simulink subsystem "Day2_Scenario_1"  (R2024a)
settings: Solver=VariableStepAuto  StartTime=0.0  StopTime=10.0  RelTol=1e-3
libraries: CarMaker4SL x2
settings Model: Creator=junhyung.cha  LastModifiedBy=User

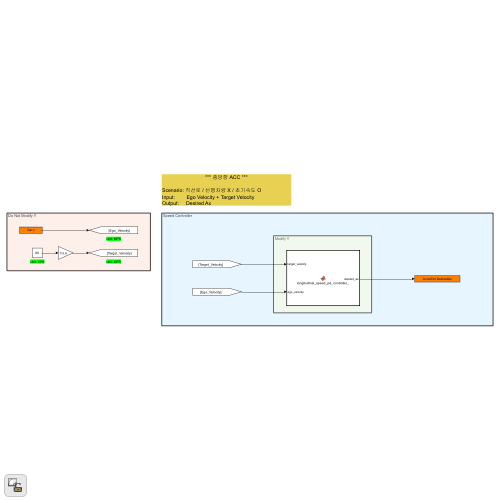
[thumbnail: Simulink's stored preview of the top-level diagram]
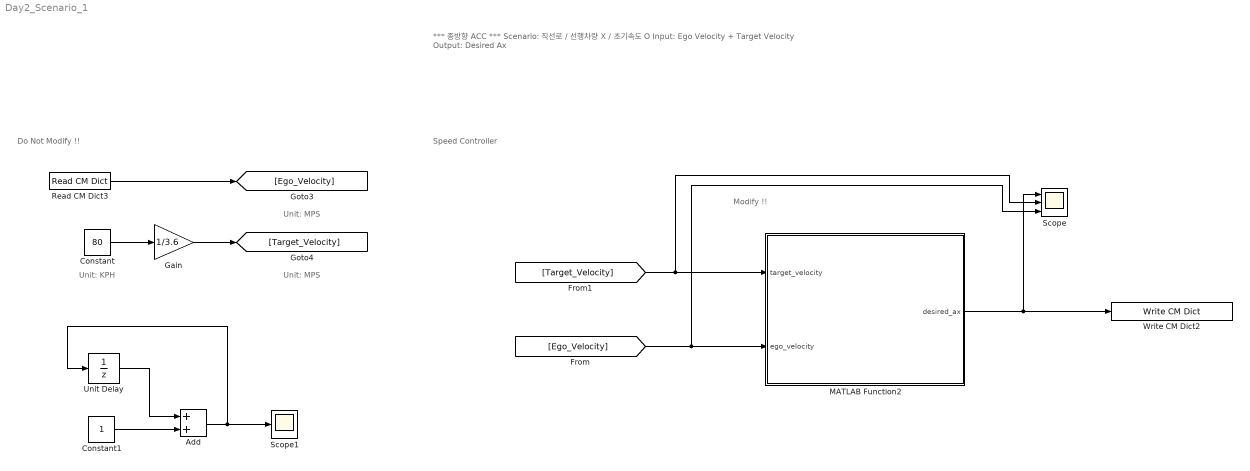
== system Day2_Scenario_1 ==
  note: Unit: KPH
  note: *** 종방향 ACC ***
      |
      | Scenario: 직선로 / 선행차량 X / 초기속도 O
      | Input: Ego Velocity + Target Velocity
      | Output: Desired Ax
  note: Do Not Modify !!
  note: Modify !!
  note: Speed Controller
  note: Unit: MPS
  note: Unit: MPS
  Add : Sum
  Constant : Constant  Value=80
  Constant1 : Constant
  Gain : Gain  Gain=1/3.6
  MATLAB Function2 : MATLAB Function  TreatAsAtomicUnit=on
  Read CM Dict3 : CarMaker4SL/Read CM Dict  xname=Car.v  xsync=off  xstime=Inherited
  Scope : Scope  NumInputPorts=3
  Scope1 : Scope
  Unit Delay : UnitDelay  SampleTime=-1  HasFrameUpgradeWarning=on
  Write CM Dict2 : CarMaker4SL/Write CM Dict  xname=AccelCtrl.DesiredAx  xsync=off
  wires:
  MATLAB Function2/1(desired_ax) -> Write CM Dict2/1, Scope/1
  [Target_Velocity] -> MATLAB Function2/1(target_velocity), Scope/2
  Constant/1 -> Gain/1
  [Ego_Velocity] -> MATLAB Function2/2(ego_velocity), Scope/3
  Read CM Dict3/1 -> [Ego_Velocity]
  Gain/1 -> [Target_Velocity]
  Unit Delay/1 -> Add/1
  Add/1 -> Unit Delay/1, Scope1/1
  Constant1/1 -> Add/2

== matlab function Day2_Scenario_1/MATLAB Function2 ==
  settings: updateMethod=DISCRETE  sampleTime=0.05
  data: target_velocity input; desired_ax output; ego_velocity input
function desired_ax = longitudinal_speed_pd_controller_(target_velocity, ego_velocity)
    %PD 제어기를 이용해서 v를 구하고, 이걸로 a를 구하기


    persistent prev_error
    persistent initialized
    dt = 0.001;

    Kp = 0.5;
    Kd = 0.1;

    if(isempty(initialized))
        prev_error = 0;
        initialized = true;
    end
    
    error = target_velocity - ego_velocity;
    deriative = (error - prev_error) / dt;


    %PD 제어기
    desired_ax = Kp*error + Kd*deriative;

    prev_error = error;


end
